simulink model "npc_controller"  (R2022a)
settings: Solver=FixedStepDiscrete  StartTime=0.0  StopTime=20  RelTol=1e-3  EnableMultiTasking=on
undefined symbols (not defined in the file): CAN_O_INT, CANA_BASE, Down, GPTRIP1SEL, GPTRIP2SEL, GPTRIP3SEL, Tsw, TZ1, TZ2, TZ3, Up, V2G_en
libraries: simulink x171, hdlsllib x90, c2802xlib x46, c2837xDlib x19, c280xlib x12, canmsglib x9, c2838xlib x8, idelinklib_common x5, c2806xlib x2, slpidlib x2, c28004xlib x2, c281xlib x2
(part 42 of 55)

== system npc_controller/CONTROL/STATE-MACHINE/CPU_CONTROL_100_inv/updateSequencePhC/pol_vxn1/neg/SR ON ==
  note: EPwm10Regs.AQCSFRC.bit.CSFB = (uint16_T)(0b01);
      | EPwm11Regs.AQCSFRC.bit.CSFB = (uint16_T)(0b00);
      | EPwm10Regs.AQCSFRC.bit.CSFA = (uint16_T)(0b10);
      | EPwm11Regs.AQCSFRC.bit.CSFA = (uint16_T)(0b00);
  note: Note:A2
      |
      | Function PWM # GPIO # LAUNCHPAD PIN #
      |
      | Synci EPWM1A GPIO0 J4.40
      | EPWM1B GPIO1 J4.39
      |
      | ORPS EPMW6A GPIO10 J8.76
      | EPWM6B GPIO11 J8.75
      |
      | RELAY EPWM3A GPIO4 J4.36
      |
      | TZ GPIO62 XX
      |
      | a_s1 EPWM2A GPIO2 J4.38 XBAR_TRIP4
      | a_s2 EPWM7B GPIO13 XX
      | a_s3 EPWM2B GPIO3 J4.37
      | a_s4 EPWM7A GPIO12 XX XBAR_TRIP5
      |
      | b_s1 EPWM8B GPIO15 J8.73 XBAR_TRIP7
      | b_s2 EPWM9B GPIO17 XX
      | b_s3 EPWM8A GPIO14 J8.74
      | b_s4 EPWM9A GPIO16 J4.33 XBAR_TRIP8
      |
      | c_s1 EPWM10B GPIO19 J1.3 XBAR_TRIP9
      | c_s2 EPWM11B GPIO21 XX
      | c_s3 EPWM10A GPIO18 J1.4
      | c_s4 EPWM11A GPIO20 XX XBAR_TRIP10
  note: Note:
      | AQCSFRC
      | 0b00 - disables forced PWM
      | 0b01 - forces PWM to LOW
      | 0b10 - forces PWM to  HIGH
  Action Port : ActionPort
  Constant : Constant  Value=2  OutDataTypeStr=uint8  SampleTime=-1
  System Outputs1 : Subsystem  mask(System Outputs){ShowInLibBrowser=0}
      mask prompts: ShowInLibBrowser "Simulink:masks:CustCodeMaskParam1_MP"
      settings: CopyFcn=cccopyfcn(gcb)  OpenFcn=ccopenfcn('System Outputs Function')
      mask Help: eval('feval(''rtwprivate'',''rtwhelpview'',''rtw_sys_outputs_block'')');
      mask Display: disp('System\nOutputs');
  Out1 : Outport
  wires:
  Constant/1 -> Out1/1

== system npc_controller/CONTROL/STATE-MACHINE/CPU_CONTROL_100_inv/updateSequencePhC/pol_vxn1/pos/S3_Blanking ==
  note: Note:
      | AQCSFRC
      | 0b00 - disables forced PWM/pass through
      | 0b01 - forces PWM to LOW
      | 0b10 - forces PWM to  HIGH
  note: Note:A2
      |
      | Function PWM # GPIO # LAUNCHPAD PIN #
      |
      | Synci EPWM1A GPIO0 J4.40
      | EPWM1B GPIO1 J4.39
      |
      | ORPS EPMW6A GPIO10 J8.76
      | EPWM6B GPIO11 J8.75
      |
      | RELAY EPWM3A GPIO4 J4.36
      |
      | TZ GPIO62 XX
      |
      | a_s1 EPWM2A GPIO2 J4.38 XBAR_TRIP4
      | a_s2 EPWM7B GPIO13 XX
      | a_s3 EPWM2B GPIO3 J4.37
      | a_s4 EPWM7A GPIO12 XX XBAR_TRIP5
      |
      | b_s1 EPWM8B GPIO15 J8.73 XBAR_TRIP7
      | b_s2 EPWM9B GPIO17 XX
      | b_s3 EPWM8A GPIO14 J8.74
      | b_s4 EPWM9A GPIO16 J4.33 XBAR_TRIP8
      |
      | c_s1 EPWM10B GPIO19 J1.3 XBAR_TRIP9
      | c_s2 EPWM11B GPIO21 XX
      | c_s3 EPWM10A GPIO18 J1.4
      | c_s4 EPWM11A GPIO20 XX XBAR_TRIP10
  note: EPwm10Regs.AQCSFRC.bit.CSFB = (uint16_T)(0b00);
      | EPwm11Regs.AQCSFRC.bit.CSFB = (uint16_T)(0b10);
      | EPwm10Regs.AQCSFRC.bit.CSFA = (uint16_T)(0b01);
      | EPwm11Regs.AQCSFRC.bit.CSFA = (uint16_T)(0b01);
  Action Port : ActionPort
  Constant : Constant  OutDataTypeStr=uint8  SampleTime=-1
  System Outputs1 : Subsystem  mask(System Outputs){ShowInLibBrowser=0}
      mask prompts: ShowInLibBrowser "Simulink:masks:CustCodeMaskParam1_MP"
      settings: CopyFcn=cccopyfcn(gcb)  OpenFcn=ccopenfcn('System Outputs Function')
      mask Help: eval('feval(''rtwprivate'',''rtwhelpview'',''rtw_sys_outputs_block'')');
      mask Display: disp('System\nOutputs');
  Out1 : Outport
  wires:
  Constant/1 -> Out1/1

== system npc_controller/CONTROL/STATE-MACHINE/CPU_CONTROL_100_inv/updateSequencePhC/pol_vxn1/pos/SR Force to Low ==
  note: EPwm10Regs.AQCSFRC.bit.CSFB = (uint16_T)(0b01);
      | EPwm11Regs.AQCSFRC.bit.CSFB = (uint16_T)(0b10);
      | EPwm10Regs.AQCSFRC.bit.CSFA = (uint16_T)(0b00);
      | EPwm11Regs.AQCSFRC.bit.CSFA = (uint16_T)(0b01);
  note: Note:
      | AQCSFRC
      | 0b00 - disables forced PWM
      | 0b01 - forces PWM to LOW
      | 0b10 - forces PWM to  HIGH
  note: Note:A2
      |
      | Function PWM # GPIO # LAUNCHPAD PIN #
      |
      | Synci EPWM1A GPIO0 J4.40
      | EPWM1B GPIO1 J4.39
      |
      | ORPS EPMW6A GPIO10 J8.76
      | EPWM6B GPIO11 J8.75
      |
      | RELAY EPWM3A GPIO4 J4.36
      |
      | TZ GPIO62 XX
      |
      | a_s1 EPWM2A GPIO2 J4.38 XBAR_TRIP4
      | a_s2 EPWM7B GPIO13 XX
      | a_s3 EPWM2B GPIO3 J4.37
      | a_s4 EPWM7A GPIO12 XX XBAR_TRIP5
      |
      | b_s1 EPWM8B GPIO15 J8.73 XBAR_TRIP7
      | b_s2 EPWM9B GPIO17 XX
      | b_s3 EPWM8A GPIO14 J8.74
      | b_s4 EPWM9A GPIO16 J4.33 XBAR_TRIP8
      |
      | c_s1 EPWM10B GPIO19 J1.3 XBAR_TRIP9
      | c_s2 EPWM11B GPIO21 XX
      | c_s3 EPWM10A GPIO18 J1.4
      | c_s4 EPWM11A GPIO20 XX XBAR_TRIP10
  Action Port : ActionPort
  Constant : Constant  OutDataTypeStr=uint8  SampleTime=-1
  System Outputs2 : Subsystem  mask(System Outputs){ShowInLibBrowser=0}
      mask prompts: ShowInLibBrowser "Simulink:masks:CustCodeMaskParam1_MP"
      settings: CopyFcn=cccopyfcn(gcb)  OpenFcn=ccopenfcn('System Outputs Function')
      mask Help: eval('feval(''rtwprivate'',''rtwhelpview'',''rtw_sys_outputs_block'')');
      mask Display: disp('System\nOutputs');
  Out1 : Outport
  wires:
  Constant/1 -> Out1/1

== system npc_controller/CONTROL/STATE-MACHINE/CPU_CONTROL_100_inv/updateSequencePhC/pol_vxn1/pos/SR ON ==
  note: EPwm10Regs.AQCSFRC.bit.CSFB = (uint16_T)(0b00);
      | EPwm11Regs.AQCSFRC.bit.CSFB = (uint16_T)(0b10);
      | EPwm10Regs.AQCSFRC.bit.CSFA = (uint16_T)(0b00);
      | EPwm11Regs.AQCSFRC.bit.CSFA = (uint16_T)(0b01);
  note: Note:A2
      |
      | Function PWM # GPIO # LAUNCHPAD PIN #
      |
      | Synci EPWM1A GPIO0 J4.40
      | EPWM1B GPIO1 J4.39
      |
      | ORPS EPMW6A GPIO10 J8.76
      | EPWM6B GPIO11 J8.75
      |
      | RELAY EPWM3A GPIO4 J4.36
      |
      | TZ GPIO62 XX
      |
      | a_s1 EPWM2A GPIO2 J4.38 XBAR_TRIP4
      | a_s2 EPWM7B GPIO13 XX
      | a_s3 EPWM2B GPIO3 J4.37
      | a_s4 EPWM7A GPIO12 XX XBAR_TRIP5
      |
      | b_s1 EPWM8B GPIO15 J8.73 XBAR_TRIP7
      | b_s2 EPWM9B GPIO17 XX
      | b_s3 EPWM8A GPIO14 J8.74
      | b_s4 EPWM9A GPIO16 J4.33 XBAR_TRIP8
      |
      | c_s1 EPWM10B GPIO19 J1.3 XBAR_TRIP9
      | c_s2 EPWM11B GPIO21 XX
      | c_s3 EPWM10A GPIO18 J1.4
      | c_s4 EPWM11A GPIO20 XX XBAR_TRIP10
  note: Note:
      | AQCSFRC
      | 0b00 - disables forced PWM/pass through
      | 0b01 - forces PWM to LOW
      | 0b10 - forces PWM to  HIGH
  Action Port : ActionPort
  Constant : Constant  OutDataTypeStr=uint8  SampleTime=-1
  System Outputs1 : Subsystem  mask(System Outputs){ShowInLibBrowser=0}
      mask prompts: ShowInLibBrowser "Simulink:masks:CustCodeMaskParam1_MP"
      settings: CopyFcn=cccopyfcn(gcb)  OpenFcn=ccopenfcn('System Outputs Function')
      mask Help: eval('feval(''rtwprivate'',''rtwhelpview'',''rtw_sys_outputs_block'')');
      mask Display: disp('System\nOutputs');
  Out1 : Outport
  wires:
  Constant/1 -> Out1/1

== system npc_controller/CONTROL/STATE-MACHINE/CPU_CONTROL_100_inv/updateSequencePhC/pol_vxn1/zero/System Outputs1 ==

== system npc_controller/CONTROL/STATE-MACHINE/CPU_CONTROL_100_inv/updateSequencePhC/pol_vxn2/neg/System Outputs1 ==

== system npc_controller/CONTROL/STATE-MACHINE/CPU_CONTROL_100_inv/updateSequencePhC/pol_vxn2/pos/System Outputs1 ==

== system npc_controller/CONTROL/STATE-MACHINE/CPU_CONTROL_100_inv/updateSequencePhC/pol_vxn2/pos/System Outputs2 ==

== system npc_controller/CONTROL/STATE-MACHINE/CPU_CONTROL_100_inv/updateSequencePhC/pol_vxn2/zero/System Outputs1 ==

== system npc_controller/CONTROL/STATE-MACHINE/CPU_CONTROL_100_inv/updateSequencePhC1/pol_final1/prot/System Outputs ==

== system npc_controller/CONTROL/STATE-MACHINE/CPU_CONTROL_100_inv/updateSequencePhC1/pol_vxn1/neg/SR OFF ==
  note: EPwm10Regs.AQCSFRC.bit.CSFB = (uint16_T)(0b01);
      | EPwm11Regs.AQCSFRC.bit.CSFB = (uint16_T)(0b00);
      | EPwm10Regs.AQCSFRC.bit.CSFA = (uint16_T)(0b10);
      | EPwm11Regs.AQCSFRC.bit.CSFA = (uint16_T)(0b01);
  note: Note:
      | AQCSFRC
      | 0b00 - disables forced PWM
      | 0b01 - forces PWM to LOW
      | 0b10 - forces PWM to  HIGH
  note: Note:A2
      |
      | Function PWM # GPIO # LAUNCHPAD PIN #
      |
      | Synci EPWM1A GPIO0 J4.40
      | EPWM1B GPIO1 J4.39
      |
      | ORPS EPMW6A GPIO10 J8.76
      | EPWM6B GPIO11 J8.75
      |
      | RELAY EPWM3A GPIO4 J4.36
      |
      | TZ GPIO62 XX
      |
      | a_s1 EPWM2A GPIO2 J4.38 XBAR_TRIP4
      | a_s2 EPWM7B GPIO13 XX
      | a_s3 EPWM2B GPIO3 J4.37
      | a_s4 EPWM7A GPIO12 XX XBAR_TRIP5
      |
      | b_s1 EPWM8B GPIO15 J8.73 XBAR_TRIP7
      | b_s2 EPWM9B GPIO17 XX
      | b_s3 EPWM8A GPIO14 J8.74
      | b_s4 EPWM9A GPIO16 J4.33 XBAR_TRIP8
      |
      | c_s1 EPWM10B GPIO19 J1.3 XBAR_TRIP9
      | c_s2 EPWM11B GPIO21 XX
      | c_s3 EPWM10A GPIO18 J1.4
      | c_s4 EPWM11A GPIO20 XX XBAR_TRIP10
  Action Port : ActionPort
  Constant : Constant  Value=2  OutDataTypeStr=uint8  SampleTime=-1
  System Outputs1 : Subsystem  mask(System Outputs){ShowInLibBrowser=0}
      mask prompts: ShowInLibBrowser "Simulink:masks:CustCodeMaskParam1_MP"
      settings: CopyFcn=cccopyfcn(gcb)  OpenFcn=ccopenfcn('System Outputs Function')
      mask Help: eval('feval(''rtwprivate'',''rtwhelpview'',''rtw_sys_outputs_block'')');
      mask Display: disp('System\nOutputs');
  Out1 : Outport
  wires:
  Constant/1 -> Out1/1

== system npc_controller/CONTROL/STATE-MACHINE/CPU_CONTROL_100_inv/updateSequencePhC1/pol_vxn1/neg/SR ON ==
  note: EPwm10Regs.AQCSFRC.bit.CSFB = (uint16_T)(0b01);
      | EPwm11Regs.AQCSFRC.bit.CSFB = (uint16_T)(0b00);
      | EPwm10Regs.AQCSFRC.bit.CSFA = (uint16_T)(0b10);
      | EPwm11Regs.AQCSFRC.bit.CSFA = (uint16_T)(0b00);
  note: Note:A2
      |
      | Function PWM # GPIO # LAUNCHPAD PIN #
      |
      | Synci EPWM1A GPIO0 J4.40
      | EPWM1B GPIO1 J4.39
      |
      | ORPS EPMW6A GPIO10 J8.76
      | EPWM6B GPIO11 J8.75
      |
      | RELAY EPWM3A GPIO4 J4.36
      |
      | TZ GPIO62 XX
      |
      | a_s1 EPWM2A GPIO2 J4.38 XBAR_TRIP4
      | a_s2 EPWM7B GPIO13 XX
      | a_s3 EPWM2B GPIO3 J4.37
      | a_s4 EPWM7A GPIO12 XX XBAR_TRIP5
      |
      | b_s1 EPWM8B GPIO15 J8.73 XBAR_TRIP7
      | b_s2 EPWM9B GPIO17 XX
      | b_s3 EPWM8A GPIO14 J8.74
      | b_s4 EPWM9A GPIO16 J4.33 XBAR_TRIP8
      |
      | c_s1 EPWM10B GPIO19 J1.3 XBAR_TRIP9
      | c_s2 EPWM11B GPIO21 XX
      | c_s3 EPWM10A GPIO18 J1.4
      | c_s4 EPWM11A GPIO20 XX XBAR_TRIP10
  note: Note:
      | AQCSFRC
      | 0b00 - disables forced PWM
      | 0b01 - forces PWM to LOW
      | 0b10 - forces PWM to  HIGH
  Action Port : ActionPort
  Constant : Constant  Value=2  OutDataTypeStr=uint8  SampleTime=-1
  System Outputs1 : Subsystem  mask(System Outputs){ShowInLibBrowser=0}
      mask prompts: ShowInLibBrowser "Simulink:masks:CustCodeMaskParam1_MP"
      settings: CopyFcn=cccopyfcn(gcb)  OpenFcn=ccopenfcn('System Outputs Function')
      mask Help: eval('feval(''rtwprivate'',''rtwhelpview'',''rtw_sys_outputs_block'')');
      mask Display: disp('System\nOutputs');
  Out1 : Outport
  wires:
  Constant/1 -> Out1/1

== system npc_controller/CONTROL/STATE-MACHINE/CPU_CONTROL_100_inv/updateSequencePhC1/pol_vxn1/pos/SR Force to Low ==
  note: EPwm10Regs.AQCSFRC.bit.CSFB = (uint16_T)(0b01);
      | EPwm11Regs.AQCSFRC.bit.CSFB = (uint16_T)(0b10);
      | EPwm10Regs.AQCSFRC.bit.CSFA = (uint16_T)(0b00);
      | EPwm11Regs.AQCSFRC.bit.CSFA = (uint16_T)(0b01);
  note: Note:
      | AQCSFRC
      | 0b00 - disables forced PWM
      | 0b01 - forces PWM to LOW
      | 0b10 - forces PWM to  HIGH
  note: Note:A2
      |
      | Function PWM # GPIO # LAUNCHPAD PIN #
      |
      | Synci EPWM1A GPIO0 J4.40
      | EPWM1B GPIO1 J4.39
      |
      | ORPS EPMW6A GPIO10 J8.76
      | EPWM6B GPIO11 J8.75
      |
      | RELAY EPWM3A GPIO4 J4.36
      |
      | TZ GPIO62 XX
      |
      | a_s1 EPWM2A GPIO2 J4.38 XBAR_TRIP4
      | a_s2 EPWM7B GPIO13 XX
      | a_s3 EPWM2B GPIO3 J4.37
      | a_s4 EPWM7A GPIO12 XX XBAR_TRIP5
      |
      | b_s1 EPWM8B GPIO15 J8.73 XBAR_TRIP7
      | b_s2 EPWM9B GPIO17 XX
      | b_s3 EPWM8A GPIO14 J8.74
      | b_s4 EPWM9A GPIO16 J4.33 XBAR_TRIP8
      |
      | c_s1 EPWM10B GPIO19 J1.3 XBAR_TRIP9
      | c_s2 EPWM11B GPIO21 XX
      | c_s3 EPWM10A GPIO18 J1.4
      | c_s4 EPWM11A GPIO20 XX XBAR_TRIP10
  Action Port : ActionPort
  Constant : Constant  OutDataTypeStr=uint8  SampleTime=-1
  System Outputs2 : Subsystem  mask(System Outputs){ShowInLibBrowser=0}
      mask prompts: ShowInLibBrowser "Simulink:masks:CustCodeMaskParam1_MP"
      settings: CopyFcn=cccopyfcn(gcb)  OpenFcn=ccopenfcn('System Outputs Function')
      mask Help: eval('feval(''rtwprivate'',''rtwhelpview'',''rtw_sys_outputs_block'')');
      mask Display: disp('System\nOutputs');
  Out1 : Outport
  wires:
  Constant/1 -> Out1/1

== system npc_controller/CONTROL/STATE-MACHINE/CPU_CONTROL_100_inv/updateSequencePhC1/pol_vxn1/pos/SR ON ==
  note: EPwm10Regs.AQCSFRC.bit.CSFB = (uint16_T)(0b00);
      | EPwm11Regs.AQCSFRC.bit.CSFB = (uint16_T)(0b10);
      | EPwm10Regs.AQCSFRC.bit.CSFA = (uint16_T)(0b00);
      | EPwm11Regs.AQCSFRC.bit.CSFA = (uint16_T)(0b01);
  note: Note:A2
      |
      | Function PWM # GPIO # LAUNCHPAD PIN #
      |
      | Synci EPWM1A GPIO0 J4.40
      | EPWM1B GPIO1 J4.39
      |
      | ORPS EPMW6A GPIO10 J8.76
      | EPWM6B GPIO11 J8.75
      |
      | RELAY EPWM3A GPIO4 J4.36
      |
      | TZ GPIO62 XX
      |
      | a_s1 EPWM2A GPIO2 J4.38 XBAR_TRIP4
      | a_s2 EPWM7B GPIO13 XX
      | a_s3 EPWM2B GPIO3 J4.37
      | a_s4 EPWM7A GPIO12 XX XBAR_TRIP5
      |
      | b_s1 EPWM8B GPIO15 J8.73 XBAR_TRIP7
      | b_s2 EPWM9B GPIO17 XX
      | b_s3 EPWM8A GPIO14 J8.74
      | b_s4 EPWM9A GPIO16 J4.33 XBAR_TRIP8
      |
      | c_s1 EPWM10B GPIO19 J1.3 XBAR_TRIP9
      | c_s2 EPWM11B GPIO21 XX
      | c_s3 EPWM10A GPIO18 J1.4
      | c_s4 EPWM11A GPIO20 XX XBAR_TRIP10
  note: Note:
      | AQCSFRC
      | 0b00 - disables forced PWM/pass through
      | 0b01 - forces PWM to LOW
      | 0b10 - forces PWM to  HIGH
  Action Port : ActionPort
  Constant : Constant  OutDataTypeStr=uint8  SampleTime=-1
  System Outputs1 : Subsystem  mask(System Outputs){ShowInLibBrowser=0}
      mask prompts: ShowInLibBrowser "Simulink:masks:CustCodeMaskParam1_MP"
      settings: CopyFcn=cccopyfcn(gcb)  OpenFcn=ccopenfcn('System Outputs Function')
      mask Help: eval('feval(''rtwprivate'',''rtwhelpview'',''rtw_sys_outputs_block'')');
      mask Display: disp('System\nOutputs');
  Out1 : Outport
  wires:
  Constant/1 -> Out1/1

== system npc_controller/CONTROL/STATE-MACHINE/CPU_CONTROL_100_inv/updateSequencePhC1/pol_vxn1/zero/System Outputs1 ==

== system npc_controller/CONTROL/STATE-MACHINE/CPU_CONTROL_100_inv/updateSequencePhC1/pol_vxn2/neg/System Outputs1 ==

== system npc_controller/CONTROL/STATE-MACHINE/CPU_CONTROL_100_inv/updateSequencePhC1/pol_vxn2/pos/System Outputs1 ==

== system npc_controller/CONTROL/STATE-MACHINE/CPU_CONTROL_100_inv/updateSequencePhC1/pol_vxn2/pos/System Outputs2 ==

== system npc_controller/CONTROL/STATE-MACHINE/CPU_CONTROL_100_inv/updateSequencePhC1/pol_vxn2/zero/System Outputs1 ==

== system npc_controller/CONTROL/STATE-MACHINE/CPU_CONTROL_200_A2_precharge_pfc_ok2/configGrid/FORCE_TZ/1P/ALL_LEGS ==
  note: Note:
      | TZCCTL
      | 0b00 - High impedance
      | 0b01 - Force to HIGH
      | 0b10 - Force to LOW
      | 0b11 - Do nothing
      |
      | AQCSFRC
      | 0b00 - disables forced PWM
      | 0b01 - forces PWM to LOW
      | 0b10 - forces PWM to  HIGH
      |
      | TZFRC.bit.OST
      | 0b0 - Do nothing
      | 0b1 - Force TZ
  note: EALLOW;
      |
      | /*Force TZ*/
      | EPwm6Regs. TZFRC.bit.OST = 0b0; //do nothing
      | EPwm7Regs. TZFRC.bit.OST = 0b0;
      | EPwm8Regs. TZFRC.bit.OST = 0b0;
      | EPwm9Regs. TZFRC.bit.OST = 0b0;
      | EPwm10Regs. TZFRC.bit.OST = 0b0;
      | EPwm11Regs. TZFRC.bit.OST = 0b0;
      |
      | EDIS;
      |
      | //change ref for leg B and legC
  Action Port : ActionPort
  System Outputs2 : Subsystem  mask(System Outputs){ShowInLibBrowser=0}
      mask prompts: ShowInLibBrowser "Simulink:masks:CustCodeMaskParam1_MP"
      settings: CopyFcn=cccopyfcn(gcb)  OpenFcn=ccopenfcn('System Outputs Function')
      mask Help: eval('feval(''rtwprivate'',''rtwhelpview'',''rtw_sys_outputs_block'')');
      mask Display: disp('System\nOutputs');

== system npc_controller/CONTROL/STATE-MACHINE/CPU_CONTROL_200_A2_precharge_pfc_ok2/configGrid/FORCE_TZ/1P/LEG_A ==
  note: EALLOW;
      |
      | /*Force TZ*/
      | EPwm6Regs. TZFRC.bit.OST = 0b0; //do nothing
      | EPwm7Regs. TZFRC.bit.OST = 0b0;
      | EPwm8Regs. TZFRC.bit.OST = 0b1;
      | EPwm9Regs. TZFRC.bit.OST = 0b1;
      | EPwm10Regs. TZFRC.bit.OST = 0b1;
      | EPwm11Regs. TZFRC.bit.OST = 0b1;
      |
      | EDIS;
  note: Note:
      | TZCCTL
      | 0b00 - High impedance
      | 0b01 - Force to HIGH
      | 0b10 - Force to LOW
      | 0b11 - Do nothing
      |
      | AQCSFRC
      | 0b00 - disables forced PWM
      | 0b01 - forces PWM to LOW
      | 0b10 - forces PWM to  HIGH
      |
      | TZFRC.bit.OST
      | 0b0 - Do nothing
      | 0b1 - Force TZ
  Action Port : ActionPort
  System Outputs2 : Subsystem  mask(System Outputs){ShowInLibBrowser=0}
      mask prompts: ShowInLibBrowser "Simulink:masks:CustCodeMaskParam1_MP"
      settings: CopyFcn=cccopyfcn(gcb)  OpenFcn=ccopenfcn('System Outputs Function')
      mask Help: eval('feval(''rtwprivate'',''rtwhelpview'',''rtw_sys_outputs_block'')');
      mask Display: disp('System\nOutputs');

== system npc_controller/CONTROL/STATE-MACHINE/CPU_CONTROL_200_A2_precharge_pfc_ok2/configGrid/FORCE_TZ/1P/LEG_B ==
  note: Note:
      | TZCCTL
      | 0b00 - High impedance
      | 0b01 - Force to HIGH
      | 0b10 - Force to LOW
      | 0b11 - Do nothing
      |
      | AQCSFRC
      | 0b00 - disables forced PWM
      | 0b01 - forces PWM to LOW
      | 0b10 - forces PWM to  HIGH
      |
      | TZFRC.bit.OST
      | 0b0 - Do nothing
      | 0b1 - Force TZ
  note: EALLOW;
      |
      | /*Force TZ*/
      | EPwm6Regs. TZFRC.bit.OST = 0b1; //do nothing
      | EPwm7Regs. TZFRC.bit.OST = 0b1;
      | EPwm8Regs. TZFRC.bit.OST = 0b0;
      | EPwm9Regs. TZFRC.bit.OST = 0b0;
      | EPwm10Regs. TZFRC.bit.OST = 0b1;
      | EPwm11Regs. TZFRC.bit.OST = 0b1;
      |
      | EDIS;
  Action Port : ActionPort
  System Outputs2 : Subsystem  mask(System Outputs){ShowInLibBrowser=0}
      mask prompts: ShowInLibBrowser "Simulink:masks:CustCodeMaskParam1_MP"
      settings: CopyFcn=cccopyfcn(gcb)  OpenFcn=ccopenfcn('System Outputs Function')
      mask Help: eval('feval(''rtwprivate'',''rtwhelpview'',''rtw_sys_outputs_block'')');
      mask Display: disp('System\nOutputs');

== system npc_controller/CONTROL/STATE-MACHINE/CPU_CONTROL_200_A2_precharge_pfc_ok2/configGrid/FORCE_TZ/1P/LEG_C ==
  note: EALLOW;
      |
      | /*Force TZ*/
      | EPwm6Regs. TZFRC.bit.OST = 0b1; //do nothing
      | EPwm7Regs. TZFRC.bit.OST = 0b1;
      | EPwm8Regs. TZFRC.bit.OST = 0b1;
      | EPwm9Regs. TZFRC.bit.OST = 0b1;
      | EPwm10Regs. TZFRC.bit.OST = 0b0;
      | EPwm11Regs. TZFRC.bit.OST = 0b0;
      |
      | EDIS;
  note: Note:
      | TZCCTL
      | 0b00 - High impedance
      | 0b01 - Force to HIGH
      | 0b10 - Force to LOW
      | 0b11 - Do nothing
      |
      | AQCSFRC
      | 0b00 - disables forced PWM
      | 0b01 - forces PWM to LOW
      | 0b10 - forces PWM to  HIGH
      |
      | TZFRC.bit.OST
      | 0b0 - Do nothing
      | 0b1 - Force TZ
  Action Port : ActionPort
  System Outputs2 : Subsystem  mask(System Outputs){ShowInLibBrowser=0}
      mask prompts: ShowInLibBrowser "Simulink:masks:CustCodeMaskParam1_MP"
      settings: CopyFcn=cccopyfcn(gcb)  OpenFcn=ccopenfcn('System Outputs Function')
      mask Help: eval('feval(''rtwprivate'',''rtwhelpview'',''rtw_sys_outputs_block'')');
      mask Display: disp('System\nOutputs');

== system npc_controller/CONTROL/STATE-MACHINE/CPU_CONTROL_200_A2_precharge_pfc_ok2/configGrid/FORCE_TZ/3P3W/System Outputs2 ==

== system npc_controller/CONTROL/STATE-MACHINE/CPU_CONTROL_200_A2_precharge_pfc_ok2/updateCalib/done/RESET_TZ/System Outputs2 ==

== system npc_controller/CONTROL/STATE-MACHINE/CPU_CONTROL_200_A2_precharge_pfc_ok2/updatePll3p/PLL/SRF_PLL/Integrator ==
  PI Out : Inport  OutDataTypeStr=single
  Accumulation : Subsystem  TreatAsAtomicUnit=on
  Add : Sum  AccumDataTypeStr=single
  Compare To Constant : simulink/Logic and Bit Operations/Compare To Constant  relop=>=  const=2*pi  OutDataTypeStr=boolean
  If : If  IfExpression=u1
  Merge : Merge
  Product : Product  OutDataTypeStr=single
  Reset Integrator : Subsystem  TreatAsAtomicUnit=on
  Ts : Constant  Value=Tsw  OutDataTypeStr=single
  Unit Delay : UnitDelay  SampleTime=-1  HasFrameUpgradeWarning=on
  wt : Outport
  wires:
  PI Out/1 -> Product/1
  Ts/1 -> Product/2
  Product/1 -> Add/1
  Add/1 -> Accumulation/1(In1), Compare To Constant/1
  Compare To Constant/1 -> If/1
  If/1 -> Reset Integrator/Action
  If/2 -> Accumulation/Action
  Reset Integrator/1(Out) -> Merge/1
  Accumulation/1(Out) -> Merge/2
  Merge/1 -> Unit Delay/1
  Unit Delay/1 -> wt/1, Add/2

== system npc_controller/CONTROL/STATE-MACHINE/CPU_CONTROL_200_A2_precharge_pfc_ok2/updatePll3p/PLL/SRF_PLL/PI ==
  Vq : Inport
  Ki : Gain  Gain=200
  Ki1 : Gain  Commented=on  Gain=200
  Kp : Gain  Gain=0.5
  Kp1 : Gain  Commented=on  Gain=0.5
  Sum : Sum  Inputs=|++
  Sum1 : Sum  Inputs=+|+
  Ts/2 : Gain  Gain=Tsw/2
  Unit Delay : UnitDelay  SampleTime=-1  HasFrameUpgradeWarning=on
  PI Out : Outport
  wires:
  Ts/2/1 -> Sum/1
  Sum1/1 -> PI Out/1
  Ki/1 -> Ts/2/1
  Vq/1 -> Ki/1, Kp/1  "Vq"
  Unit Delay/1 -> Sum/2
  Kp/1 -> Sum1/1
  Sum/1 -> Sum1/2, Unit Delay/1

== system npc_controller/CONTROL/STATE-MACHINE/CPU_CONTROL_200_A2_precharge_pfc_ok2/updatePll3p/PLL/SRF_PLL/Subsystem1 ==
  x[n] : Inport
  1 - Lambda : Gain  Gain=1 - 0.98
  Delay : Delay  DelayLength=1
  Gain{,1..7} (8 alike) : Gain  Commented=on  Gain=1/8
  Lambda : Gain  Gain=0.98
  Memory{,1..6} (7 alike) : Memory  Commented=on  InheritSampleTime=on
  Sum{,1..6} (7 alike) : Sum  Commented=on  Inputs=++|
  Sum7 : Sum  Inputs=|++
  y[n] : Outport
  wires:
  Sum7/1 -> y[n]/1, Delay/1
  Delay/1 -> Lambda/1
  1 - Lambda/1 -> Sum7/1
  x[n]/1 -> 1 - Lambda/1
  Lambda/1 -> Sum7/2
  Gain7/1 -> Sum6/1
  Sum5/1 -> Sum6/2
  Memory6/1 -> Gain7/1
  Memory5/1 -> Gain6/1, Memory6/1
  Sum4/1 -> Sum5/2
  Gain6/1 -> Sum5/1
  Gain5/1 -> Sum4/1
  Sum3/1 -> Sum4/2
  Memory4/1 -> Gain5/1, Memory5/1
  Memory3/1 -> Gain4/1, Memory4/1
  Sum2/1 -> Sum3/2
  Gain4/1 -> Sum3/1
  Gain3/1 -> Sum2/1
  Sum1/1 -> Sum2/2
  Gain2/1 -> Sum1/1
  Sum/1 -> Sum1/2
  Gain1/1 -> Sum/1
  Gain/1 -> Sum/2
  Memory2/1 -> Gain3/1, Memory3/1
  Memory1/1 -> Gain2/1, Memory2/1
  Memory/1 -> Gain1/1, Memory1/1

== system npc_controller/CONTROL/STATE-MACHINE/CPU_CONTROL_200_A2_precharge_pfc_ok2/updatePll3p/PLL/SRF_PLL/abc to dq ==
  note: wt
  note: wt
  note: wt
  a : Inport
  b : Inport  Port=2
  c : Inport  Port=3
  wt : Inport  Port=4
  (wt+120) : Sum  Inputs=|++
  (wt-120) : Sum  Inputs=|+-
  2pi_3 : Constant  Value=2*pi/3
  Add3 : Sum  Inputs=+++
  Cos3 : Trigonometry  Operator=cos
  Cos4 : Trigonometry  Operator=cos
  Cos5 : Trigonometry  Operator=cos
  Product5 : Product
  Product6 : Product
  Product7 : Product
  q1 : Gain  Gain=2/3
  q : Outport
  wires:
  [a] -> Product5/1
  Cos3/1 -> Product5/2
  wt/1 -> (wt+120)/1, (wt-120)/1, Cos3/1
  [ph] -> (wt+120)/2
  Product7/1 -> Add3/3
  a/1 -> [a]
  (wt+120)/1 -> Cos5/1
  Product6/1 -> Add3/2
  c/1 -> [c]
  [ph] -> (wt-120)/2
  (wt-120)/1 -> Cos4/1
  [b] -> Product6/1
  Cos4/1 -> Product6/2
  Product5/1 -> Add3/1
  Cos5/1 -> Product7/2
  b/1 -> [b]
  Add3/1 -> q1/1
  [c] -> Product7/1
  q1/1 -> q/1
  2pi_3/1 -> [ph]

== system npc_controller/CONTROL/STATE-MACHINE/CPU_CONTROL_200_A2_precharge_pfc_ok2/updatePll3p/PLL/Subsystem/Initialize at Zero Crossing ==
  In1 : Inport
  Trigger : TriggerPort  VariantControl=Variant
  OR : Logic  Operator=OR  IconShape=distinctive  AllPortsSameDT=off  OutDataTypeStr=boolean
  Unit Delay : UnitDelay  SampleTime=-1  HasFrameUpgradeWarning=on
  Out1 : Outport  InitialOutput=0  VectorParamsAs1DForOutWhenUnconnected=off
  wires:
  OR/1 -> Out1/1, Unit Delay/1
  Unit Delay/1 -> OR/2
  In1/1 -> OR/1

== system npc_controller/CONTROL/STATE-MACHINE/CPU_CONTROL_200_A2_precharge_pfc_ok2/updateSequencePhA/pol_final1/prot/System Outputs ==

== system npc_controller/CONTROL/STATE-MACHINE/CPU_CONTROL_200_A2_precharge_pfc_ok2/updateSequencePhA/pol_vxn1/neg/System Outputs1 ==

== system npc_controller/CONTROL/STATE-MACHINE/CPU_CONTROL_200_A2_precharge_pfc_ok2/updateSequencePhA/pol_vxn1/pos/System Outputs1 ==

== system npc_controller/CONTROL/STATE-MACHINE/CPU_CONTROL_200_A2_precharge_pfc_ok2/updateSequencePhA/pol_vxn1/zero/System Outputs1 ==

== system npc_controller/CONTROL/STATE-MACHINE/CPU_CONTROL_200_A2_precharge_pfc_ok2/updateSequencePhB/pol_final1/prot/System Outputs ==

== system npc_controller/CONTROL/STATE-MACHINE/CPU_CONTROL_200_A2_precharge_pfc_ok2/updateSequencePhB/pol_vxn1/neg/System Outputs1 ==

== system npc_controller/CONTROL/STATE-MACHINE/CPU_CONTROL_200_A2_precharge_pfc_ok2/updateSequencePhB/pol_vxn1/pos/System Outputs1 ==

== system npc_controller/CONTROL/STATE-MACHINE/CPU_CONTROL_200_A2_precharge_pfc_ok2/updateSequencePhB/pol_vxn1/zero/System Outputs1 ==

== system npc_controller/CONTROL/STATE-MACHINE/CPU_CONTROL_200_A2_precharge_pfc_ok2/updateSequencePhC/pol_final1/prot/System Outputs ==

== system npc_controller/CONTROL/STATE-MACHINE/CPU_CONTROL_200_A2_precharge_pfc_ok2/updateSequencePhC/pol_vxn1/neg/System Outputs1 ==

== system npc_controller/CONTROL/STATE-MACHINE/CPU_CONTROL_200_A2_precharge_pfc_ok2/updateSequencePhC/pol_vxn1/pos/System Outputs1 ==

== system npc_controller/CONTROL/STATE-MACHINE/CPU_CONTROL_200_A2_precharge_pfc_ok2/updateSequencePhC/pol_vxn1/zero/System Outputs1 ==

== system npc_controller/CONTROL/STATE-MACHINE/CPU_CONTROL_200_A2_precharge_pfc_ok2_OL SS/configGrid/FORCE_TZ/1P/ALL_LEGS ==
  note: Note:
      | TZCCTL
      | 0b00 - High impedance
      | 0b01 - Force to HIGH
      | 0b10 - Force to LOW
      | 0b11 - Do nothing
      |
      | AQCSFRC
      | 0b00 - disables forced PWM
      | 0b01 - forces PWM to LOW
      | 0b10 - forces PWM to  HIGH
      |
      | TZFRC.bit.OST
      | 0b0 - Do nothing
      | 0b1 - Force TZ
  note: EALLOW;
      |
      | /*Force TZ*/
      | EPwm6Regs. TZFRC.bit.OST = 0b0; //do nothing
      | EPwm7Regs. TZFRC.bit.OST = 0b0;
      | EPwm8Regs. TZFRC.bit.OST = 0b0;
      | EPwm9Regs. TZFRC.bit.OST = 0b0;
      | EPwm10Regs. TZFRC.bit.OST = 0b0;
      | EPwm11Regs. TZFRC.bit.OST = 0b0;
      |
      | EDIS;
      |
      | //change ref for leg B and legC
  Action Port : ActionPort
  System Outputs2 : Subsystem  mask(System Outputs){ShowInLibBrowser=0}
      mask prompts: ShowInLibBrowser "Simulink:masks:CustCodeMaskParam1_MP"
      settings: CopyFcn=cccopyfcn(gcb)  OpenFcn=ccopenfcn('System Outputs Function')
      mask Help: eval('feval(''rtwprivate'',''rtwhelpview'',''rtw_sys_outputs_block'')');
      mask Display: disp('System\nOutputs');

== system npc_controller/CONTROL/STATE-MACHINE/CPU_CONTROL_200_A2_precharge_pfc_ok2_OL SS/configGrid/FORCE_TZ/1P/LEG_A ==
  note: EALLOW;
      |
      | /*Force TZ*/
      | EPwm6Regs. TZFRC.bit.OST = 0b0; //do nothing
      | EPwm7Regs. TZFRC.bit.OST = 0b0;
      | EPwm8Regs. TZFRC.bit.OST = 0b1;
      | EPwm9Regs. TZFRC.bit.OST = 0b1;
      | EPwm10Regs. TZFRC.bit.OST = 0b1;
      | EPwm11Regs. TZFRC.bit.OST = 0b1;
      |
      | EDIS;
  note: Note:
      | TZCCTL
      | 0b00 - High impedance
      | 0b01 - Force to HIGH
      | 0b10 - Force to LOW
      | 0b11 - Do nothing
      |
      | AQCSFRC
      | 0b00 - disables forced PWM
      | 0b01 - forces PWM to LOW
      | 0b10 - forces PWM to  HIGH
      |
      | TZFRC.bit.OST
      | 0b0 - Do nothing
      | 0b1 - Force TZ
  Action Port : ActionPort
  System Outputs2 : Subsystem  mask(System Outputs){ShowInLibBrowser=0}
      mask prompts: ShowInLibBrowser "Simulink:masks:CustCodeMaskParam1_MP"
      settings: CopyFcn=cccopyfcn(gcb)  OpenFcn=ccopenfcn('System Outputs Function')
      mask Help: eval('feval(''rtwprivate'',''rtwhelpview'',''rtw_sys_outputs_block'')');
      mask Display: disp('System\nOutputs');

== system npc_controller/CONTROL/STATE-MACHINE/CPU_CONTROL_200_A2_precharge_pfc_ok2_OL SS/configGrid/FORCE_TZ/1P/LEG_B ==
  note: Note:
      | TZCCTL
      | 0b00 - High impedance
      | 0b01 - Force to HIGH
      | 0b10 - Force to LOW
      | 0b11 - Do nothing
      |
      | AQCSFRC
      | 0b00 - disables forced PWM
      | 0b01 - forces PWM to LOW
      | 0b10 - forces PWM to  HIGH
      |
      | TZFRC.bit.OST
      | 0b0 - Do nothing
      | 0b1 - Force TZ
  note: EALLOW;
      |
      | /*Force TZ*/
      | EPwm6Regs. TZFRC.bit.OST = 0b1; //do nothing
      | EPwm7Regs. TZFRC.bit.OST = 0b1;
      | EPwm8Regs. TZFRC.bit.OST = 0b0;
      | EPwm9Regs. TZFRC.bit.OST = 0b0;
      | EPwm10Regs. TZFRC.bit.OST = 0b1;
      | EPwm11Regs. TZFRC.bit.OST = 0b1;
      |
      | EDIS;
  Action Port : ActionPort
  System Outputs2 : Subsystem  mask(System Outputs){ShowInLibBrowser=0}
      mask prompts: ShowInLibBrowser "Simulink:masks:CustCodeMaskParam1_MP"
      settings: CopyFcn=cccopyfcn(gcb)  OpenFcn=ccopenfcn('System Outputs Function')
      mask Help: eval('feval(''rtwprivate'',''rtwhelpview'',''rtw_sys_outputs_block'')');
      mask Display: disp('System\nOutputs');

== system npc_controller/CONTROL/STATE-MACHINE/CPU_CONTROL_200_A2_precharge_pfc_ok2_OL SS/configGrid/FORCE_TZ/1P/LEG_C ==
  note: EALLOW;
      |
      | /*Force TZ*/
      | EPwm6Regs. TZFRC.bit.OST = 0b1; //do nothing
      | EPwm7Regs. TZFRC.bit.OST = 0b1;
      | EPwm8Regs. TZFRC.bit.OST = 0b1;
      | EPwm9Regs. TZFRC.bit.OST = 0b1;
      | EPwm10Regs. TZFRC.bit.OST = 0b0;
      | EPwm11Regs. TZFRC.bit.OST = 0b0;
      |
      | EDIS;
  note: Note:
      | TZCCTL
      | 0b00 - High impedance
      | 0b01 - Force to HIGH
      | 0b10 - Force to LOW
      | 0b11 - Do nothing
      |
      | AQCSFRC
      | 0b00 - disables forced PWM
      | 0b01 - forces PWM to LOW
      | 0b10 - forces PWM to  HIGH
      |
      | TZFRC.bit.OST
      | 0b0 - Do nothing
      | 0b1 - Force TZ
  Action Port : ActionPort
  System Outputs2 : Subsystem  mask(System Outputs){ShowInLibBrowser=0}
      mask prompts: ShowInLibBrowser "Simulink:masks:CustCodeMaskParam1_MP"
      settings: CopyFcn=cccopyfcn(gcb)  OpenFcn=ccopenfcn('System Outputs Function')
      mask Help: eval('feval(''rtwprivate'',''rtwhelpview'',''rtw_sys_outputs_block'')');
      mask Display: disp('System\nOutputs');

== system npc_controller/CONTROL/STATE-MACHINE/CPU_CONTROL_200_A2_precharge_pfc_ok2_OL SS/configGrid/FORCE_TZ/3P3W/System Outputs2 ==

== system npc_controller/CONTROL/STATE-MACHINE/CPU_CONTROL_200_A2_precharge_pfc_ok2_OL SS/updateCalib/done/RESET_TZ/System Outputs2 ==

== system npc_controller/CONTROL/STATE-MACHINE/CPU_CONTROL_200_A2_precharge_pfc_ok2_OL SS/updatePll3p/PLL/SRF_PLL/Integrator ==
  PI Out : Inport  OutDataTypeStr=single
  Accumulation : Subsystem  TreatAsAtomicUnit=on
  Add : Sum  AccumDataTypeStr=single
  Compare To Constant : simulink/Logic and Bit Operations/Compare To Constant  relop=>=  const=2*pi  OutDataTypeStr=boolean
  If : If  IfExpression=u1
  Merge : Merge
  Product : Product  OutDataTypeStr=single
  Reset Integrator : Subsystem  TreatAsAtomicUnit=on
  Ts : Constant  Value=Tsw  OutDataTypeStr=single
  Unit Delay : UnitDelay  SampleTime=-1  HasFrameUpgradeWarning=on
  wt : Outport
  wires:
  PI Out/1 -> Product/1
  Ts/1 -> Product/2
  Product/1 -> Add/1
  Add/1 -> Accumulation/1(In1), Compare To Constant/1
  Compare To Constant/1 -> If/1
  If/1 -> Reset Integrator/Action
  If/2 -> Accumulation/Action
  Reset Integrator/1(Out) -> Merge/1
  Accumulation/1(Out) -> Merge/2
  Merge/1 -> Unit Delay/1
  Unit Delay/1 -> wt/1, Add/2

== system npc_controller/CONTROL/STATE-MACHINE/CPU_CONTROL_200_A2_precharge_pfc_ok2_OL SS/updatePll3p/PLL/SRF_PLL/PI ==
  Vq : Inport
  Ki : Gain  Gain=200
  Ki1 : Gain  Commented=on  Gain=200
  Kp : Gain  Gain=0.5
  Kp1 : Gain  Commented=on  Gain=0.5
  Sum : Sum  Inputs=|++
  Sum1 : Sum  Inputs=+|+
  Ts/2 : Gain  Gain=Tsw/2
  Unit Delay : UnitDelay  SampleTime=-1  HasFrameUpgradeWarning=on
  PI Out : Outport
  wires:
  Ts/2/1 -> Sum/1
  Sum1/1 -> PI Out/1
  Ki/1 -> Ts/2/1
  Vq/1 -> Ki/1, Kp/1  "Vq"
  Unit Delay/1 -> Sum/2
  Kp/1 -> Sum1/1
  Sum/1 -> Sum1/2, Unit Delay/1

== system npc_controller/CONTROL/STATE-MACHINE/CPU_CONTROL_200_A2_precharge_pfc_ok2_OL SS/updatePll3p/PLL/SRF_PLL/Subsystem1 ==
  x[n] : Inport
  1 - Lambda : Gain  Gain=1 - 0.98
  Delay : Delay  DelayLength=1
  Gain{,1..7} (8 alike) : Gain  Commented=on  Gain=1/8
  Lambda : Gain  Gain=0.98
  Memory{,1..6} (7 alike) : Memory  Commented=on  InheritSampleTime=on
  Sum{,1..6} (7 alike) : Sum  Commented=on  Inputs=++|
  Sum7 : Sum  Inputs=|++
  y[n] : Outport
  wires:
  Sum7/1 -> y[n]/1, Delay/1
  Delay/1 -> Lambda/1
  1 - Lambda/1 -> Sum7/1
  x[n]/1 -> 1 - Lambda/1
  Lambda/1 -> Sum7/2
  Gain7/1 -> Sum6/1
  Sum5/1 -> Sum6/2
  Memory6/1 -> Gain7/1
  Memory5/1 -> Gain6/1, Memory6/1
  Sum4/1 -> Sum5/2
  Gain6/1 -> Sum5/1
  Gain5/1 -> Sum4/1
  Sum3/1 -> Sum4/2
  Memory4/1 -> Gain5/1, Memory5/1
  Memory3/1 -> Gain4/1, Memory4/1
  Sum2/1 -> Sum3/2
  Gain4/1 -> Sum3/1
  Gain3/1 -> Sum2/1
  Sum1/1 -> Sum2/2
  Gain2/1 -> Sum1/1
  Sum/1 -> Sum1/2
  Gain1/1 -> Sum/1
  Gain/1 -> Sum/2
  Memory2/1 -> Gain3/1, Memory3/1
  Memory1/1 -> Gain2/1, Memory2/1
  Memory/1 -> Gain1/1, Memory1/1

== system npc_controller/CONTROL/STATE-MACHINE/CPU_CONTROL_200_A2_precharge_pfc_ok2_OL SS/updatePll3p/PLL/SRF_PLL/abc to dq ==
  note: wt
  note: wt
  note: wt
  a : Inport
  b : Inport  Port=2
  c : Inport  Port=3
  wt : Inport  Port=4
  (wt+120) : Sum  Inputs=|++
  (wt-120) : Sum  Inputs=|+-
  2pi_3 : Constant  Value=2*pi/3
  Add3 : Sum  Inputs=+++
  Cos3 : Trigonometry  Operator=cos
  Cos4 : Trigonometry  Operator=cos
  Cos5 : Trigonometry  Operator=cos
  Product5 : Product
  Product6 : Product
  Product7 : Product
  q1 : Gain  Gain=2/3
  q : Outport
  wires:
  [a] -> Product5/1
  Cos3/1 -> Product5/2
  wt/1 -> (wt+120)/1, (wt-120)/1, Cos3/1
  [ph] -> (wt+120)/2
  Product7/1 -> Add3/3
  a/1 -> [a]
  (wt+120)/1 -> Cos5/1
  Product6/1 -> Add3/2
  c/1 -> [c]
  [ph] -> (wt-120)/2
  (wt-120)/1 -> Cos4/1
  [b] -> Product6/1
  Cos4/1 -> Product6/2
  Product5/1 -> Add3/1
  Cos5/1 -> Product7/2
  b/1 -> [b]
  Add3/1 -> q1/1
  [c] -> Product7/1
  q1/1 -> q/1
  2pi_3/1 -> [ph]

== system npc_controller/CONTROL/STATE-MACHINE/CPU_CONTROL_200_A2_precharge_pfc_ok2_OL SS/updatePll3p/PLL/Subsystem/Initialize at Zero Crossing ==
  In1 : Inport
  Trigger : TriggerPort  VariantControl=Variant
  OR : Logic  Operator=OR  IconShape=distinctive  AllPortsSameDT=off  OutDataTypeStr=boolean
  Unit Delay : UnitDelay  SampleTime=-1  HasFrameUpgradeWarning=on
  Out1 : Outport  InitialOutput=0  VectorParamsAs1DForOutWhenUnconnected=off
  wires:
  OR/1 -> Out1/1, Unit Delay/1
  Unit Delay/1 -> OR/2
  In1/1 -> OR/1

== system npc_controller/CONTROL/STATE-MACHINE/CPU_CONTROL_200_A2_precharge_pfc_ok2_OL SS/updateSequencePhA/pol_final1/prot/System Outputs ==

== system npc_controller/CONTROL/STATE-MACHINE/CPU_CONTROL_200_A2_precharge_pfc_ok2_OL SS/updateSequencePhA/pol_vxn1/neg/System Outputs1 ==

== system npc_controller/CONTROL/STATE-MACHINE/CPU_CONTROL_200_A2_precharge_pfc_ok2_OL SS/updateSequencePhA/pol_vxn1/pos/System Outputs1 ==

== system npc_controller/CONTROL/STATE-MACHINE/CPU_CONTROL_200_A2_precharge_pfc_ok2_OL SS/updateSequencePhA/pol_vxn1/zero/System Outputs1 ==

== system npc_controller/CONTROL/STATE-MACHINE/CPU_CONTROL_200_A2_precharge_pfc_ok2_OL SS/updateSequencePhB/pol_final1/prot/System Outputs ==

== system npc_controller/CONTROL/STATE-MACHINE/CPU_CONTROL_200_A2_precharge_pfc_ok2_OL SS/updateSequencePhB/pol_vxn1/neg/System Outputs1 ==

== system npc_controller/CONTROL/STATE-MACHINE/CPU_CONTROL_200_A2_precharge_pfc_ok2_OL SS/updateSequencePhB/pol_vxn1/pos/System Outputs1 ==

== system npc_controller/CONTROL/STATE-MACHINE/CPU_CONTROL_200_A2_precharge_pfc_ok2_OL SS/updateSequencePhB/pol_vxn1/zero/System Outputs1 ==

== system npc_controller/CONTROL/STATE-MACHINE/CPU_CONTROL_200_A2_precharge_pfc_ok2_OL SS/updateSequencePhC/pol_final1/prot/System Outputs ==

== system npc_controller/CONTROL/STATE-MACHINE/CPU_CONTROL_200_A2_precharge_pfc_ok2_OL SS/updateSequencePhC/pol_vxn1/neg/System Outputs1 ==

== system npc_controller/CONTROL/STATE-MACHINE/CPU_CONTROL_200_A2_precharge_pfc_ok2_OL SS/updateSequencePhC/pol_vxn1/pos/System Outputs1 ==

== system npc_controller/CONTROL/STATE-MACHINE/CPU_CONTROL_200_A2_precharge_pfc_ok2_OL SS/updateSequencePhC/pol_vxn1/zero/System Outputs1 ==

== system npc_controller/CONTROL/STATE-MACHINE/CPU_CONTROL_200_Vpk/configGrid/FORCE_TZ/1P/ALL_LEGS ==
  note: Note:
      | TZCCTL
      | 0b00 - High impedance
      | 0b01 - Force to HIGH
      | 0b10 - Force to LOW
      | 0b11 - Do nothing
      |
      | AQCSFRC
      | 0b00 - disables forced PWM
      | 0b01 - forces PWM to LOW
      | 0b10 - forces PWM to  HIGH
      |
      | TZFRC.bit.OST
      | 0b0 - Do nothing
      | 0b1 - Force TZ
  note: EALLOW;
      |
      | /*Force TZ*/
      | EPwm6Regs. TZFRC.bit.OST = 0b0; //do nothing
      | EPwm7Regs. TZFRC.bit.OST = 0b0;
      | EPwm8Regs. TZFRC.bit.OST = 0b0;
      | EPwm9Regs. TZFRC.bit.OST = 0b0;
      | EPwm10Regs. TZFRC.bit.OST = 0b0;
      | EPwm11Regs. TZFRC.bit.OST = 0b0;
      |
      | EDIS;
      |
      | //change ref for leg B and legC
  Action Port : ActionPort
  System Outputs2 : Subsystem  mask(System Outputs){ShowInLibBrowser=0}
      mask prompts: ShowInLibBrowser "Simulink:masks:CustCodeMaskParam1_MP"
      settings: CopyFcn=cccopyfcn(gcb)  OpenFcn=ccopenfcn('System Outputs Function')
      mask Help: eval('feval(''rtwprivate'',''rtwhelpview'',''rtw_sys_outputs_block'')');
      mask Display: disp('System\nOutputs');

== system npc_controller/CONTROL/STATE-MACHINE/CPU_CONTROL_200_Vpk/configGrid/FORCE_TZ/1P/LEG_A ==
  note: EALLOW;
      |
      | /*Force TZ*/
      | EPwm6Regs. TZFRC.bit.OST = 0b0; //do nothing
      | EPwm7Regs. TZFRC.bit.OST = 0b0;
      | EPwm8Regs. TZFRC.bit.OST = 0b1;
      | EPwm9Regs. TZFRC.bit.OST = 0b1;
      | EPwm10Regs. TZFRC.bit.OST = 0b1;
      | EPwm11Regs. TZFRC.bit.OST = 0b1;
      |
      | EDIS;
  note: Note:
      | TZCCTL
      | 0b00 - High impedance
      | 0b01 - Force to HIGH
      | 0b10 - Force to LOW
      | 0b11 - Do nothing
      |
      | AQCSFRC
      | 0b00 - disables forced PWM
      | 0b01 - forces PWM to LOW
      | 0b10 - forces PWM to  HIGH
      |
      | TZFRC.bit.OST
      | 0b0 - Do nothing
      | 0b1 - Force TZ
  Action Port : ActionPort
  System Outputs2 : Subsystem  mask(System Outputs){ShowInLibBrowser=0}
      mask prompts: ShowInLibBrowser "Simulink:masks:CustCodeMaskParam1_MP"
      settings: CopyFcn=cccopyfcn(gcb)  OpenFcn=ccopenfcn('System Outputs Function')
      mask Help: eval('feval(''rtwprivate'',''rtwhelpview'',''rtw_sys_outputs_block'')');
      mask Display: disp('System\nOutputs');

== system npc_controller/CONTROL/STATE-MACHINE/CPU_CONTROL_200_Vpk/configGrid/FORCE_TZ/1P/LEG_B ==
  note: Note:
      | TZCCTL
      | 0b00 - High impedance
      | 0b01 - Force to HIGH
      | 0b10 - Force to LOW
      | 0b11 - Do nothing
      |
      | AQCSFRC
      | 0b00 - disables forced PWM
      | 0b01 - forces PWM to LOW
      | 0b10 - forces PWM to  HIGH
      |
      | TZFRC.bit.OST
      | 0b0 - Do nothing
      | 0b1 - Force TZ
  note: EALLOW;
      |
      | /*Force TZ*/
      | EPwm6Regs. TZFRC.bit.OST = 0b1; //do nothing
      | EPwm7Regs. TZFRC.bit.OST = 0b1;
      | EPwm8Regs. TZFRC.bit.OST = 0b0;
      | EPwm9Regs. TZFRC.bit.OST = 0b0;
      | EPwm10Regs. TZFRC.bit.OST = 0b1;
      | EPwm11Regs. TZFRC.bit.OST = 0b1;
      |
      | EDIS;
  Action Port : ActionPort
  System Outputs2 : Subsystem  mask(System Outputs){ShowInLibBrowser=0}
      mask prompts: ShowInLibBrowser "Simulink:masks:CustCodeMaskParam1_MP"
      settings: CopyFcn=cccopyfcn(gcb)  OpenFcn=ccopenfcn('System Outputs Function')
      mask Help: eval('feval(''rtwprivate'',''rtwhelpview'',''rtw_sys_outputs_block'')');
      mask Display: disp('System\nOutputs');

== system npc_controller/CONTROL/STATE-MACHINE/CPU_CONTROL_200_Vpk/configGrid/FORCE_TZ/1P/LEG_C ==
  note: EALLOW;
      |
      | /*Force TZ*/
      | EPwm6Regs. TZFRC.bit.OST = 0b1; //do nothing
      | EPwm7Regs. TZFRC.bit.OST = 0b1;
      | EPwm8Regs. TZFRC.bit.OST = 0b1;
      | EPwm9Regs. TZFRC.bit.OST = 0b1;
      | EPwm10Regs. TZFRC.bit.OST = 0b0;
      | EPwm11Regs. TZFRC.bit.OST = 0b0;
      |
      | EDIS;
  note: Note:
      | TZCCTL
      | 0b00 - High impedance
      | 0b01 - Force to HIGH
      | 0b10 - Force to LOW
      | 0b11 - Do nothing
      |
      | AQCSFRC
      | 0b00 - disables forced PWM
      | 0b01 - forces PWM to LOW
      | 0b10 - forces PWM to  HIGH
      |
      | TZFRC.bit.OST
      | 0b0 - Do nothing
      | 0b1 - Force TZ
  Action Port : ActionPort
  System Outputs2 : Subsystem  mask(System Outputs){ShowInLibBrowser=0}
      mask prompts: ShowInLibBrowser "Simulink:masks:CustCodeMaskParam1_MP"
      settings: CopyFcn=cccopyfcn(gcb)  OpenFcn=ccopenfcn('System Outputs Function')
      mask Help: eval('feval(''rtwprivate'',''rtwhelpview'',''rtw_sys_outputs_block'')');
      mask Display: disp('System\nOutputs');

== system npc_controller/CONTROL/STATE-MACHINE/CPU_CONTROL_200_Vpk/configGrid/FORCE_TZ/3P3W/System Outputs2 ==

== system npc_controller/CONTROL/STATE-MACHINE/CPU_CONTROL_200_Vpk/updateCalib/done/RESET_TZ/System Outputs2 ==

== system npc_controller/CONTROL/STATE-MACHINE/CPU_CONTROL_200_Vpk/updatePll3p/PLL/SRF_PLL/Integrator ==
  PI Out : Inport  OutDataTypeStr=single
  Accumulation : Subsystem  TreatAsAtomicUnit=on
  Add : Sum  AccumDataTypeStr=single
  Compare To Constant : simulink/Logic and Bit Operations/Compare To Constant  relop=>=  const=2*pi  OutDataTypeStr=boolean
  If : If  IfExpression=u1
  Merge : Merge
  Product : Product  OutDataTypeStr=single
  Reset Integrator : Subsystem  TreatAsAtomicUnit=on
  Ts : Constant  Value=Tsw  OutDataTypeStr=single
  Unit Delay : UnitDelay  SampleTime=-1  HasFrameUpgradeWarning=on
  wt : Outport
  wires:
  PI Out/1 -> Product/1
  Ts/1 -> Product/2
  Product/1 -> Add/1
  Add/1 -> Accumulation/1(In1), Compare To Constant/1
  Compare To Constant/1 -> If/1
  If/1 -> Reset Integrator/Action
  If/2 -> Accumulation/Action
  Reset Integrator/1(Out) -> Merge/1
  Accumulation/1(Out) -> Merge/2
  Merge/1 -> Unit Delay/1
  Unit Delay/1 -> wt/1, Add/2

== system npc_controller/CONTROL/STATE-MACHINE/CPU_CONTROL_200_Vpk/updatePll3p/PLL/SRF_PLL/PI ==
  Vq : Inport
  Ki : Gain  Gain=200
  Ki1 : Gain  Commented=on  Gain=200
  Kp : Gain  Gain=0.5
  Kp1 : Gain  Commented=on  Gain=0.5
  Sum : Sum  Inputs=|++
  Sum1 : Sum  Inputs=+|+
  Ts/2 : Gain  Gain=Tsw/2
  Unit Delay : UnitDelay  SampleTime=-1  HasFrameUpgradeWarning=on
  PI Out : Outport
  wires:
  Ts/2/1 -> Sum/1
  Sum1/1 -> PI Out/1
  Ki/1 -> Ts/2/1
  Vq/1 -> Ki/1, Kp/1  "Vq"
  Unit Delay/1 -> Sum/2
  Kp/1 -> Sum1/1
  Sum/1 -> Sum1/2, Unit Delay/1

== system npc_controller/CONTROL/STATE-MACHINE/CPU_CONTROL_200_Vpk/updatePll3p/PLL/SRF_PLL/Subsystem1 ==
  x[n] : Inport
  1 - Lambda : Gain  Gain=1 - 0.98
  Delay : Delay  DelayLength=1
  Gain{,1..7} (8 alike) : Gain  Commented=on  Gain=1/8
  Lambda : Gain  Gain=0.98
  Memory{,1..6} (7 alike) : Memory  Commented=on  InheritSampleTime=on
  Sum{,1..6} (7 alike) : Sum  Commented=on  Inputs=++|
  Sum7 : Sum  Inputs=|++
  y[n] : Outport
  wires:
  Sum7/1 -> y[n]/1, Delay/1
  Delay/1 -> Lambda/1
  1 - Lambda/1 -> Sum7/1
  x[n]/1 -> 1 - Lambda/1
  Lambda/1 -> Sum7/2
  Gain7/1 -> Sum6/1
  Sum5/1 -> Sum6/2
  Memory6/1 -> Gain7/1
  Memory5/1 -> Gain6/1, Memory6/1
  Sum4/1 -> Sum5/2
  Gain6/1 -> Sum5/1
  Gain5/1 -> Sum4/1
  Sum3/1 -> Sum4/2
  Memory4/1 -> Gain5/1, Memory5/1
  Memory3/1 -> Gain4/1, Memory4/1
  Sum2/1 -> Sum3/2
  Gain4/1 -> Sum3/1
  Gain3/1 -> Sum2/1
  Sum1/1 -> Sum2/2
  Gain2/1 -> Sum1/1
  Sum/1 -> Sum1/2
  Gain1/1 -> Sum/1
  Gain/1 -> Sum/2
  Memory2/1 -> Gain3/1, Memory3/1
  Memory1/1 -> Gain2/1, Memory2/1
  Memory/1 -> Gain1/1, Memory1/1

== system npc_controller/CONTROL/STATE-MACHINE/CPU_CONTROL_200_Vpk/updatePll3p/PLL/SRF_PLL/abc to dq ==
  note: wt
  note: wt
  note: wt
  a : Inport
  b : Inport  Port=2
  c : Inport  Port=3
  wt : Inport  Port=4
  (wt+120) : Sum  Inputs=|++
  (wt-120) : Sum  Inputs=|+-
  2pi_3 : Constant  Value=2*pi/3
  Add3 : Sum  Inputs=+++
  Cos3 : Trigonometry  Operator=cos
  Cos4 : Trigonometry  Operator=cos
  Cos5 : Trigonometry  Operator=cos
  Product5 : Product
  Product6 : Product
  Product7 : Product
  q1 : Gain  Gain=2/3
  q : Outport
  wires:
  [a] -> Product5/1
  Cos3/1 -> Product5/2
  wt/1 -> (wt+120)/1, (wt-120)/1, Cos3/1
  [ph] -> (wt+120)/2
  Product7/1 -> Add3/3
  a/1 -> [a]
  (wt+120)/1 -> Cos5/1
  Product6/1 -> Add3/2
  c/1 -> [c]
  [ph] -> (wt-120)/2
  (wt-120)/1 -> Cos4/1
  [b] -> Product6/1
  Cos4/1 -> Product6/2
  Product5/1 -> Add3/1
  Cos5/1 -> Product7/2
  b/1 -> [b]
  Add3/1 -> q1/1
  [c] -> Product7/1
  q1/1 -> q/1
  2pi_3/1 -> [ph]

== system npc_controller/CONTROL/STATE-MACHINE/CPU_CONTROL_200_Vpk/updatePll3p/PLL/Subsystem/Initialize at Zero Crossing ==
  In1 : Inport
  Trigger : TriggerPort  VariantControl=Variant
  OR : Logic  Operator=OR  IconShape=distinctive  AllPortsSameDT=off  OutDataTypeStr=boolean
  Unit Delay : UnitDelay  SampleTime=-1  HasFrameUpgradeWarning=on
  Out1 : Outport  InitialOutput=0  VectorParamsAs1DForOutWhenUnconnected=off
  wires:
  OR/1 -> Out1/1, Unit Delay/1
  Unit Delay/1 -> OR/2
  In1/1 -> OR/1

== system npc_controller/CONTROL/STATE-MACHINE/CPU_CONTROL_200_Vpk/updateSequencePhA/pol_final1/prot/System Outputs ==

== system npc_controller/CONTROL/STATE-MACHINE/CPU_CONTROL_200_Vpk/updateSequencePhA/pol_vxn1/neg/System Outputs1 ==

== system npc_controller/CONTROL/STATE-MACHINE/CPU_CONTROL_200_Vpk/updateSequencePhA/pol_vxn1/pos/System Outputs1 ==

== system npc_controller/CONTROL/STATE-MACHINE/CPU_CONTROL_200_Vpk/updateSequencePhA/pol_vxn1/pos/System Outputs2 ==

== system npc_controller/CONTROL/STATE-MACHINE/CPU_CONTROL_200_Vpk/updateSequencePhA/pol_vxn1/zero/System Outputs1 ==

== system npc_controller/CONTROL/STATE-MACHINE/CPU_CONTROL_200_Vpk/updateSequencePhB/pol_final1/prot/System Outputs ==

== system npc_controller/CONTROL/STATE-MACHINE/CPU_CONTROL_200_Vpk/updateSequencePhB/pol_vxn1/neg/System Outputs1 ==

== system npc_controller/CONTROL/STATE-MACHINE/CPU_CONTROL_200_Vpk/updateSequencePhB/pol_vxn1/pos/System Outputs1 ==

== system npc_controller/CONTROL/STATE-MACHINE/CPU_CONTROL_200_Vpk/updateSequencePhB/pol_vxn1/zero/System Outputs1 ==

== system npc_controller/CONTROL/STATE-MACHINE/CPU_CONTROL_200_Vpk/updateSequencePhC/pol_final1/prot/System Outputs ==

== system npc_controller/CONTROL/STATE-MACHINE/CPU_CONTROL_200_Vpk/updateSequencePhC/pol_vxn1/neg/System Outputs1 ==

== system npc_controller/CONTROL/STATE-MACHINE/CPU_CONTROL_200_Vpk/updateSequencePhC/pol_vxn1/pos/System Outputs1 ==

== system npc_controller/CONTROL/STATE-MACHINE/CPU_CONTROL_200_Vpk/updateSequencePhC/pol_vxn1/zero/System Outputs1 ==

== system npc_controller/CONTROL/STATE-MACHINE/CPU_CONTROL_200_inv/configGrid/FORCE_TZ/1P/ALL_LEGS ==
  note: Note:
      | TZCCTL
      | 0b00 - High impedance
      | 0b01 - Force to HIGH
      | 0b10 - Force to LOW
      | 0b11 - Do nothing
      |
      | AQCSFRC
      | 0b00 - disables forced PWM
      | 0b01 - forces PWM to LOW
      | 0b10 - forces PWM to  HIGH
      |
      | TZFRC.bit.OST
      | 0b0 - Do nothing
      | 0b1 - Force TZ
  note: EALLOW;
      |
      | /*Force TZ*/
      | EPwm6Regs. TZFRC.bit.OST = 0b0; //do nothing
      | EPwm7Regs. TZFRC.bit.OST = 0b0;
      | EPwm8Regs. TZFRC.bit.OST = 0b0;
      | EPwm9Regs. TZFRC.bit.OST = 0b0;
      | EPwm10Regs. TZFRC.bit.OST = 0b0;
      | EPwm11Regs. TZFRC.bit.OST = 0b0;
      |
      | EDIS;
      |
      | //change ref for leg B and legC
  Action Port : ActionPort
  System Outputs2 : Subsystem  mask(System Outputs){ShowInLibBrowser=0}
      mask prompts: ShowInLibBrowser "Simulink:masks:CustCodeMaskParam1_MP"
      settings: CopyFcn=cccopyfcn(gcb)  OpenFcn=ccopenfcn('System Outputs Function')
      mask Help: eval('feval(''rtwprivate'',''rtwhelpview'',''rtw_sys_outputs_block'')');
      mask Display: disp('System\nOutputs');

== system npc_controller/CONTROL/STATE-MACHINE/CPU_CONTROL_200_inv/configGrid/FORCE_TZ/1P/LEG_A ==
  note: EALLOW;
      |
      | /*Force TZ*/
      | EPwm6Regs. TZFRC.bit.OST = 0b0; //do nothing
      | EPwm7Regs. TZFRC.bit.OST = 0b0;
      | EPwm8Regs. TZFRC.bit.OST = 0b1;
      | EPwm9Regs. TZFRC.bit.OST = 0b1;
      | EPwm10Regs. TZFRC.bit.OST = 0b1;
      | EPwm11Regs. TZFRC.bit.OST = 0b1;
      |
      | EDIS;
  note: Note:
      | TZCCTL
      | 0b00 - High impedance
      | 0b01 - Force to HIGH
      | 0b10 - Force to LOW
      | 0b11 - Do nothing
      |
      | AQCSFRC
      | 0b00 - disables forced PWM
      | 0b01 - forces PWM to LOW
      | 0b10 - forces PWM to  HIGH
      |
      | TZFRC.bit.OST
      | 0b0 - Do nothing
      | 0b1 - Force TZ
  Action Port : ActionPort
  System Outputs2 : Subsystem  mask(System Outputs){ShowInLibBrowser=0}
      mask prompts: ShowInLibBrowser "Simulink:masks:CustCodeMaskParam1_MP"
      settings: CopyFcn=cccopyfcn(gcb)  OpenFcn=ccopenfcn('System Outputs Function')
      mask Help: eval('feval(''rtwprivate'',''rtwhelpview'',''rtw_sys_outputs_block'')');
      mask Display: disp('System\nOutputs');

== system npc_controller/CONTROL/STATE-MACHINE/CPU_CONTROL_200_inv/configGrid/FORCE_TZ/1P/LEG_B ==
  note: Note:
      | TZCCTL
      | 0b00 - High impedance
      | 0b01 - Force to HIGH
      | 0b10 - Force to LOW
      | 0b11 - Do nothing
      |
      | AQCSFRC
      | 0b00 - disables forced PWM
      | 0b01 - forces PWM to LOW
      | 0b10 - forces PWM to  HIGH
      |
      | TZFRC.bit.OST
      | 0b0 - Do nothing
      | 0b1 - Force TZ
  note: EALLOW;
      |
      | /*Force TZ*/
      | EPwm6Regs. TZFRC.bit.OST = 0b1; //do nothing
      | EPwm7Regs. TZFRC.bit.OST = 0b1;
      | EPwm8Regs. TZFRC.bit.OST = 0b0;
      | EPwm9Regs. TZFRC.bit.OST = 0b0;
      | EPwm10Regs. TZFRC.bit.OST = 0b1;
      | EPwm11Regs. TZFRC.bit.OST = 0b1;
      |
      | EDIS;
  Action Port : ActionPort
  System Outputs2 : Subsystem  mask(System Outputs){ShowInLibBrowser=0}
      mask prompts: ShowInLibBrowser "Simulink:masks:CustCodeMaskParam1_MP"
      settings: CopyFcn=cccopyfcn(gcb)  OpenFcn=ccopenfcn('System Outputs Function')
      mask Help: eval('feval(''rtwprivate'',''rtwhelpview'',''rtw_sys_outputs_block'')');
      mask Display: disp('System\nOutputs');

== system npc_controller/CONTROL/STATE-MACHINE/CPU_CONTROL_200_inv/configGrid/FORCE_TZ/1P/LEG_C ==
  note: EALLOW;
      |
      | /*Force TZ*/
      | EPwm6Regs. TZFRC.bit.OST = 0b1; //do nothing
      | EPwm7Regs. TZFRC.bit.OST = 0b1;
      | EPwm8Regs. TZFRC.bit.OST = 0b1;
      | EPwm9Regs. TZFRC.bit.OST = 0b1;
      | EPwm10Regs. TZFRC.bit.OST = 0b0;
      | EPwm11Regs. TZFRC.bit.OST = 0b0;
      |
      | EDIS;
  note: Note:
      | TZCCTL
      | 0b00 - High impedance
      | 0b01 - Force to HIGH
      | 0b10 - Force to LOW
      | 0b11 - Do nothing
      |
      | AQCSFRC
      | 0b00 - disables forced PWM
      | 0b01 - forces PWM to LOW
      | 0b10 - forces PWM to  HIGH
      |
      | TZFRC.bit.OST
      | 0b0 - Do nothing
      | 0b1 - Force TZ
  Action Port : ActionPort
  System Outputs2 : Subsystem  mask(System Outputs){ShowInLibBrowser=0}
      mask prompts: ShowInLibBrowser "Simulink:masks:CustCodeMaskParam1_MP"
      settings: CopyFcn=cccopyfcn(gcb)  OpenFcn=ccopenfcn('System Outputs Function')
      mask Help: eval('feval(''rtwprivate'',''rtwhelpview'',''rtw_sys_outputs_block'')');
      mask Display: disp('System\nOutputs');

== system npc_controller/CONTROL/STATE-MACHINE/CPU_CONTROL_200_inv/configGrid/FORCE_TZ/3P3W/System Outputs2 ==

== system npc_controller/CONTROL/STATE-MACHINE/CPU_CONTROL_200_inv/updateCalib/done/RESET_TZ/System Outputs1 ==

== system npc_controller/CONTROL/STATE-MACHINE/CPU_CONTROL_200_inv/updateCalib/done/RESET_TZ/System Outputs2 ==

== system npc_controller/CONTROL/STATE-MACHINE/CPU_CONTROL_200_inv/updatePll3p/PLL/SRF_PLL/Integrator ==
  PI Out : Inport  OutDataTypeStr=single
  Accumulation : Subsystem  TreatAsAtomicUnit=on
  Add : Sum  AccumDataTypeStr=single
  Compare To Constant : simulink/Logic and Bit Operations/Compare To Constant  relop=>=  const=2*pi  OutDataTypeStr=boolean
  If : If  IfExpression=u1
  Merge : Merge
  Product : Product  OutDataTypeStr=single
  Reset Integrator : Subsystem  TreatAsAtomicUnit=on
  Ts : Constant  Value=Tsw  OutDataTypeStr=single
  Unit Delay : UnitDelay  SampleTime=-1  HasFrameUpgradeWarning=on
  wt : Outport
  wires:
  PI Out/1 -> Product/1
  Ts/1 -> Product/2
  Product/1 -> Add/1
  Add/1 -> Accumulation/1(In1), Compare To Constant/1
  Compare To Constant/1 -> If/1
  If/1 -> Reset Integrator/Action
  If/2 -> Accumulation/Action
  Reset Integrator/1(Out) -> Merge/1
  Accumulation/1(Out) -> Merge/2
  Merge/1 -> Unit Delay/1
  Unit Delay/1 -> wt/1, Add/2

== system npc_controller/CONTROL/STATE-MACHINE/CPU_CONTROL_200_inv/updatePll3p/PLL/SRF_PLL/PI ==
  Vq : Inport
  Ki : Gain  Gain=200
  Ki1 : Gain  Commented=on  Gain=200
  Kp : Gain  Gain=0.5
  Kp1 : Gain  Commented=on  Gain=0.5
  Sum : Sum  Inputs=|++
  Sum1 : Sum  Inputs=+|+
  Ts/2 : Gain  Gain=Tsw/2
  Unit Delay : UnitDelay  SampleTime=-1  HasFrameUpgradeWarning=on
  PI Out : Outport
  wires:
  Ts/2/1 -> Sum/1
  Sum1/1 -> PI Out/1
  Ki/1 -> Ts/2/1
  Vq/1 -> Ki/1, Kp/1  "Vq"
  Unit Delay/1 -> Sum/2
  Kp/1 -> Sum1/1
  Sum/1 -> Sum1/2, Unit Delay/1
